simulink model "autopilota_v_15_last"  (R2022a)
settings: Solver=ode4  StartTime=0.0  StopTime=300  FixedStep=0.02  RelTol=1e-3
values from neighbouring files (symbols this model uses):
  attuatore_Amax = 20*(pi/180)    (= 0.349065850399)    [v2021_10_27_avvioSITL.m]    (also in v2021_10_27_calcoloAerodinamica.m)
  attuatore_Amin = -20*(pi/180)    (= -0.349065850399)    [v2021_10_27_avvioSITL.m]
  attuatore_Emax = 25*(pi/180)    (= 0.436332312999)    [v2021_10_27_avvioSITL.m]    (also in v2021_10_27_calcoloAerodinamica.m)
  attuatore_Emin = -25*(pi/180)    (= -0.436332312999)    [v2021_10_27_avvioSITL.m]
  attuatore_Rmax = 25*(pi/180)    (= 0.436332312999)    [v2021_10_27_avvioSITL.m]    (also in v2021_10_27_calcoloAerodinamica.m)
  attuatore_Rmin = -25*(pi/180)    (= -0.436332312999)    [v2021_10_27_avvioSITL.m]
  attuatore_Tmax = 0.99    [v2021_10_27_avvioSITL.m]
  attuatore_Tmin = 0    [v2021_10_27_avvioSITL.m]
  baccxINI = 0    [v2021_10_27_avvioSITL.m]
  baccyINI = 0    [v2021_10_27_avvioSITL.m]
  bacczINI = 0    [v2021_10_27_avvioSITL.m]
  bias = [baccxINI,baccyINI,bacczINI,bpINI,bqINI,brINI]    [v2021_10_27_avvioSITL.m]
  bpINI = 0    [v2021_10_27_avvioSITL.m]
  bqINI = 0    [v2021_10_27_avvioSITL.m]
  brINI = 0    [v2021_10_27_avvioSITL.m]
  final_h = 35    [v2021_10_27_avvioSITL.m]
  interventoA_05 = 20*0.8    (= 16)    [v2021_10_27_avvioSITL.m]
  interventoA_1 = 10    [v2021_10_27_avvioSITL.m]
  interventoE_05 = 25*0.8    (= 20)    [v2021_10_27_avvioSITL.m]
  interventoE_1 = 10    [v2021_10_27_avvioSITL.m]
  interventoT = 1*0.6    (= 0.6)    [v2021_10_27_avvioSITL.m]
  inv_A = 1    [v2021_10_27_avvioSITL.m]
  inv_comp_h = 1    [v2021_10_27_avvioSITL.m]
  inv_E = 1    [v2021_10_27_avvioSITL.m]
  inv_R = 1    [v2021_10_27_avvioSITL.m]
  inv_T = 1    [v2021_10_27_avvioSITL.m]
  K_AW_B_AP_quota = 1000    [v2021_10_27_avvioSITL.m]
  K_AW_B_becc = -250    [v2021_10_27_avvioSITL.m]
  K_AW_B_imb = 0    [v2021_10_27_avvioSITL.m]
  K_AW_B_roll = 500    [v2021_10_27_avvioSITL.m]
  K_imb_inv = -0.001306    [v2021_10_27_avvioSITL.m]
  Kd_AP_rotta = 0.995    [v2021_10_27_avvioSITL.m]
  Kd_h_app = 0.085    [v2021_10_27_avvioSITL.m]
  Kd_h_flare = 0.01    [v2021_10_27_avvioSITL.m]
  Ki_AP_quota_select = 0.01936    [v2021_10_27_avvioSITL.m]
  Ki_AP_rotta = 0.002    [v2021_10_27_avvioSITL.m]
  Ki_AP_vel = 0.025175    [v2021_10_27_avvioSITL.m]
  Ki_becch = -0.1963    [v2021_10_27_avvioSITL.m]
  Ki_h_app = 0.055    [v2021_10_27_avvioSITL.m]
  Ki_h_cruise = 0.008    [v2021_10_27_avvioSITL.m]
  Ki_h_flare = 0.07    [v2021_10_27_avvioSITL.m]
  Ki_roll = 0.004528    [v2021_10_27_avvioSITL.m]
  Kp_AP_quota_hold_h = 0.5503    [v2021_10_27_avvioSITL.m]
  Kp_AP_quota_hold_l = 0.5503    [v2021_10_27_avvioSITL.m]
  Kp_AP_quota_select = 0.02647    [v2021_10_27_avvioSITL.m]
  Kp_AP_rotta = 0.520    (= 0.52)    [v2021_10_27_avvioSITL.m]
  Kp_AP_vel = 0.132175    [v2021_10_27_avvioSITL.m]
  Kp_becch = -0.30    (= -0.3)    [v2021_10_27_avvioSITL.m]
  Kp_comp_h = 0.035    [v2021_10_27_avvioSITL.m]
  Kp_h_app_max = 0.086    [v2021_10_27_avvioSITL.m]
  Kp_h_app_min = 0.01    [v2021_10_27_avvioSITL.m]
  Kp_h_cruise = 0.04    [v2021_10_27_avvioSITL.m]
  Kp_h_flare = 0.1    [v2021_10_27_avvioSITL.m]
  Kp_imb = 0.0019415    [v2021_10_27_avvioSITL.m]
  Kp_p = 0.006913    [v2021_10_27_avvioSITL.m]
  Kp_q = -0.025    [v2021_10_27_avvioSITL.m]
  Kp_roll = 0.0718    [v2021_10_27_avvioSITL.m]
  Kp_Rotta_ATO = 4    [v2021_10_27_avvioSITL.m]
  Kp_Rotta_psi = -0.01    [v2021_10_27_avvioSITL.m]
  safe_phi = 55    [v2021_10_27_avvioSITL.m]
  safe_V = 40    [v2021_10_27_avvioSITL.m]
  Sensor_Offsets = [0,0,0]    [v2021_10_27_avvioSITL.m]
  theta_rot = 10    [v2021_10_27_avvioSITL.m]
  time_alarm_SAFE = 300    [v2021_10_27_avvioSITL.m]
  tsamp = 0.02    [v2021_10_27_avvioSITL.m]
  V_max = 35    [v2021_10_27_avvioSITL.m]
  V_stall = 15    [v2021_10_27_avvioSITL.m]
  vd_ini = 0    [v2021_10_27_avvioSITL.m]
  vel_wp1_al = 25    [v2021_10_27_avvioSITL.m]
  vel_wp2_al = 20    [v2021_10_27_avvioSITL.m]
undefined symbols (not defined in the file or in its folder): DiscIntNeverNeededParam, Newton, Q1B, R1B, Raphson, t_AP
libraries: simulink_extras x36, slpidlib x8, dspsigops x4, aerolibtransform2sys x2, aerolibtransform2 x2, cstblocks x1, simulink x1
(part 1 of 8)
settings Model: Creator=39339  LastModifiedBy=mvisc
settings SolverCC: AlgebraicLoopSolver=TrustRegion
settings DataIOCC: ReturnWorkspaceOutputs=off
settings DebuggingCC: ParameterPrecisionLossMsg=none  UnconnectedInputMsg=warning  UnconnectedOutputMsg=warning  UnconnectedLineMsg=warning  SFMachineParentedDataDiag=warning  ArithmeticOperatorsInVariantConditions=warning
settings ModelReferenceCC: ModelReferenceNumInstancesAllowed=Single
settings SFSimCC: SimUseLocalCustomCode=off  CustomCodeUndefinedFunction=UseInterfaceOnly
settings RTWCC: RTWUseLocalCustomCode=off  DLArmComputeVersion=19.05
settings CodeAppCC: StateflowObjectComments=on

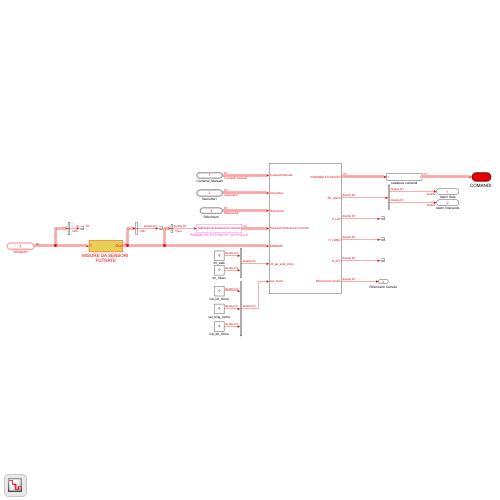
[thumbnail: Simulink's stored preview of the top-level diagram]
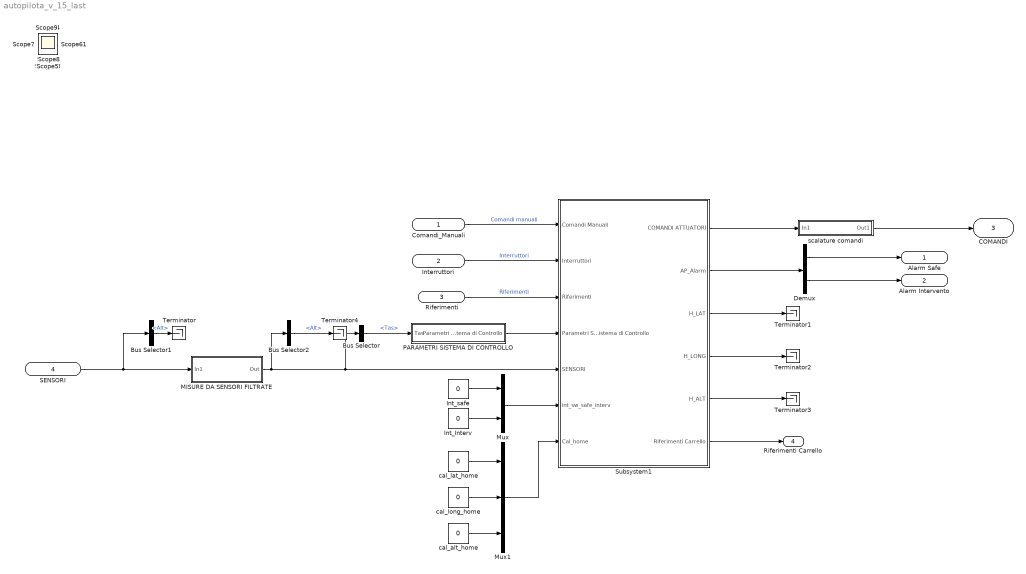
== system autopilota_v_15_last ==
  Comandi_Manuali : Inport  OutDataTypeStr=Bus: slBus4_manuali  SampleTime=[0.02,0]
  "Interruttori " : Inport  Port=2  OutDataTypeStr=Bus: slBus5_Interruttori  SampleTime=[0.02,0]
  Riferimenti : Inport  Port=3  OutDataTypeStr=Bus: slBus6_Riferimenti  SampleTime=[0.02,0]
  SENSORI : Inport  Port=4  OutDataTypeStr=Bus: slBus8_sensori2  SampleTime=[0.02,0]
  Bus Selector : BusSelector  OutputSignals=Tas
  Bus Selector1 : BusSelector  OutputSignals=Alt
  Bus Selector2 : BusSelector  OutputSignals=Alt
  Demux : Demux  Outputs=2
  Int_Interv : Constant  Value=0  SampleTime=t_AP
  Int_safe : Constant  Value=0  SampleTime=t_AP
  MISURE DA SENSORI FILTRATE : Subsystem
  Mux : Mux  Inputs=2
  Mux1 : Mux  Inputs=3
  PARAMETRI SISTEMA DI CONTROLLO : Subsystem
  Subsystem1 : Subsystem
  Terminator{,1..4} (5 alike) : Terminator
  cal_alt_home : Constant  Value=0  SampleTime=t_AP
  cal_lat_home : Constant  Value=0  SampleTime=t_AP
  cal_long_home : Constant  Value=0  SampleTime=t_AP
  "scalature comandi " : Subsystem
  Alarm Safe : Outport  OutDataTypeStr=double  PortDimensions=1  SampleTime=[0.02,0]  VectorParamsAs1DForOutWhenUnconnected=off
  Alarm Intervento : Outport  Port=2  OutDataTypeStr=double  PortDimensions=1  SampleTime=[0.02,0]  VectorParamsAs1DForOutWhenUnconnected=off
  "COMANDI " : Outport  Port=3  OutDataTypeStr=Bus: slBus8_comandi  SampleTime=[0.02,0]  VectorParamsAs1DForOutWhenUnconnected=off  LockScale=on
  Riferimenti Carrello : Outport  Port=4  VectorParamsAs1DForOutWhenUnconnected=off
  Scope{,1..11} (12 alike) : Scope
  wires:
  cal_long_home/1 -> Mux1/2
  Comandi_Manuali/1 -> Subsystem1/1(Comandi Manuali)  "Comandi manuali"
  Bus Selector/1 -> PARAMETRI SISTEMA DI CONTROLLO/1(Tas)  "<Tas>"
  "Interruttori "/1 -> Subsystem1/2("Interruttori ")  "Interruttori"
  PARAMETRI SISTEMA DI CONTROLLO/1(Parametri Sistema di Controllo) -> Subsystem1/4(Parametri Sistema di Controllo)
  Subsystem1/3(H_LAT) -> Terminator1/1
  Demux/1 -> Alarm Safe/1
  Subsystem1/5(H_ALT) -> Terminator3/1
  cal_lat_home/1 -> Mux1/1
  Int_safe/1 -> Mux/1
  Riferimenti/1 -> Subsystem1/3(Riferimenti)  "Riferimenti"
  Mux1/1 -> Subsystem1/7(Cal_home)
  cal_alt_home/1 -> Mux1/3
  Int_Interv/1 -> Mux/2
  Demux/2 -> Alarm Intervento/1
  Subsystem1/4(H_LONG) -> Terminator2/1
  Subsystem1/2(AP_Alarm) -> Demux/1
  Mux/1 -> Subsystem1/6(int_sw_safe_interv)
  SENSORI/1 -> MISURE DA SENSORI FILTRATE/1(In1), Bus Selector1/1
  MISURE DA SENSORI FILTRATE/1(Out) -> Bus Selector/1, Subsystem1/5(SENSORI), Bus Selector2/1
  "scalature comandi "/1(Out1) -> "COMANDI "/1
  Bus Selector2/1 -> Terminator4/1  "<Alt>"
  Bus Selector1/1 -> Terminator/1  "<Alt>"
  Subsystem1/6(Riferimenti Carrello) -> Riferimenti Carrello/1
  Subsystem1/1(COMANDI ATTUATORI) -> "scalature comandi "/1(In1)

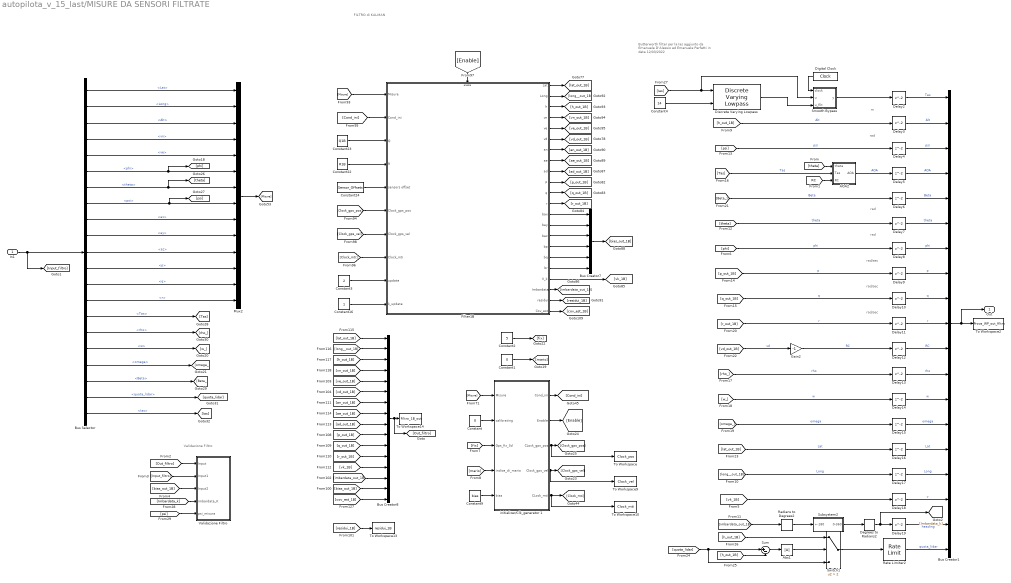
== system autopilota_v_15_last/MISURE DA SENSORI FILTRATE ==
  note: Validazione Filtro
  note: Butterworth filter per la Ias aggiunto da Emanuele D'Alessio ed Emanuele Perfetti in data 12/03/2022
  note: rad/sec
  note: rad/sec
  note: rad
  note: rad/sec
  note: FILTRO di KALMAN
  note: m
  note: rad
  note: rad
  In1 : Inport
  AOA2 : Subsystem
  Abs1 : Abs  SaturateOnIntegerOverflow=off
  Bus Creator1 : BusCreator  Inputs=19  OutDataTypeStr=Bus: slBus7_sensori
  Bus Creator7 : BusCreator  Inputs=6
  Bus Creator8 : BusCreator  Inputs=16
  Bus Selector : BusSelector  OutputSignals=Lat,Long,Alt,vn,ve,phi,theta,psi,ax,ay,az,p,q,r,Tas,rho,w,omega,Beta,quota_lidar,Ias
  Constant : Constant  Value=0
  Constant1 : Constant  Value=0
  Constant16 : Constant
  Constant2 : Constant  Value=5
  Constant22 : Constant  Value=R1B
  Constant23 : Constant  Value=Q1B
  Constant24 : Constant  Value=Sensor_Offsets
  Constant3 : Constant  Value=2
  Constant4 : Constant  Value=14
  Constant9 : Constant  Value=bias
  Degrees to Radians2 : simulink_extras/Transformations/Degrees to Radians
  Delay{2..19} (18 alike) : Delay
  Digital Clock : DigitalClock  SampleTime=0.02
  Discrete Varying Lowpass : cstblocks/Linear Parameter Varying/Discrete Varying Lowpass  N=2  w0=0  Ts=0.02
      settings: SourceProductBaseCode=CT
  Filter1B : Subsystem
  Gain2 : Gain  Gain=-1
  Mux2 : Mux  Inputs=14
  Radians to Degrees2 : simulink_extras/Transformations/Radians to Degrees
  Rate Limiter2 : RateLimiter  RisingSlewLimit=6  FallingSlewLimit=-6  SampleTimeMode=inherited
  Smooth Bypass : MATLAB Function  TreatAsAtomicUnit=on
  Subsystem2 : Subsystem
  Sum : Sum  Inputs=|+-
  Switch1 : Switch  Criteria=u2 > Threshold  Threshold=2  SaturateOnIntegerOverflow=off  InputSameDT=off
  To Workspace : ToWorkspace  VariableName=Clock_pos  SaveFormat=Timeseries  SampleTime=-1
  To Workspace10 : ToWorkspace  VariableName=Clock_mti  SaveFormat=Timeseries  SampleTime=-1
  To Workspace13 : ToWorkspace  VariableName=residui_1B  SaveFormat=Structure With Time  SampleTime=-1
  To Workspace14 : ToWorkspace  VariableName=Filtro_1B_out  SaveFormat=Timeseries  SampleTime=-1
  To Workspace2 : ToWorkspace  VariableName=Prova_WP_out_filtro  SaveFormat=Timeseries  SampleTime=-1
  To Workspace9 : ToWorkspace  VariableName=Clock_vel  SaveFormat=Timeseries  SampleTime=-1
  Validazione Filtro : Subsystem
  initializer/Clk_generator 1 : Subsystem
  Out : Outport  OutDataTypeStr=Bus: slBus7_sensori  VectorParamsAs1DForOutWhenUnconnected=off
  wires:
  Constant16/1 -> Filter1B/10(k_update)
  [Misure] -> initializer/Clk_generator 1/1(Misure)
  Delay14/1 -> Bus Creator1/13  "w"
  [Clock_gps_vel] -> Filter1B/7(Clock_gps_vel)
  Filter1B/21(residui) -> [residui_1B]
  Bus Selector/14 -> Mux2/14  "<r>"
  Filter1B/11(q) -> [q_out_1B]
  Filter1B/9(ad) -> [ad_out_1B]
  Filter1B/16(bp) -> Bus Creator7/4
  Gain2/1 -> Delay12/1  "RC"
  Filter1B/17(bq) -> Bus Creator7/5
  [long__out_1B] -> Bus Creator8/2
  [Clock_mti] -> Filter1B/8(Clock_mti)
  [mario] -> initializer/Clk_generator 1/4(indice_di_mario)
  Bus Creator7/1 -> [bias_out_1B]
  [h_out_1B] -> Bus Creator8/3
  [an_out_1B] -> Bus Creator8/7
  [Clock_gps_pos] -> Filter1B/6(Clock_gps_pos)
  Bus Selector/10 -> Mux2/10  "<ay>"
  [ad_out_1B] -> Bus Creator8/9
  Filter1B/5(ve) -> [ve_out_1B]
  Filter1B/3(h) -> [h_out_1B]
  [ae_out_1B] -> Bus Creator8/8
  Bus Creator8/1 -> [Out_filtro], To Workspace14/1
  Bus Selector/13 -> Mux2/13  "<q>"
  Constant3/1 -> Filter1B/9(update)
  [h_out_1B] -> Delay3/1  "Alt"
  Constant9/1 -> initializer/Clk_generator 1/5(bias)
  Filter1B/4(vn) -> [vn_out_1B]
  [lat_out_1B] -> Delay16/1  "Lat"
  [w_] -> Delay14/1  "w"
  Constant24/1 -> Filter1B/5(sensors offset)
  [Cond_ini] -> Filter1B/2(Cond_ini)
  Constant2/1 -> [fix]
  Filter1B/13(bax) -> Bus Creator7/1
  Filter1B/8(ae) -> [ae_out_1B]
  Filter1B/15(baz) -> Bus Creator7/3
  Delay19/1 -> Bus Creator1/18  "heading"
  [Misure] -> Filter1B/1(Misure)
  Delay9/1 -> Bus Creator1/8  "p"
  Filter1B/12(r) -> [r_out_1B]
  [vd_out_1B] -> Gain2/1  "vd"
  Filter1B/10(p) -> [p_out_1B]
  [cov_est_1B] -> Bus Creator8/16
  initializer/Clk_generator 1/5(CLock_mti) -> To Workspace10/1, [Clock_mti]
  Filter1B/6(vd) -> [vd_out_1B]
  Filter1B/22(Cov_est) -> [cov_est_1B]
  initializer/Clk_generator 1/2(Enable) -> [Enable]
  [vn_out_1B] -> Bus Creator8/4
  [imbardata_out_1B] -> Bus Creator8/14
  [vd_out_1B] -> Bus Creator8/6
  [Beta_] -> Delay6/1  "Beta"
  Delay6/1 -> Bus Creator1/5  "Beta"
  [rho_] -> Delay13/1  "rho"
  Mux2/1 -> [Misure]
  initializer/Clk_generator 1/4("Clock_gps_vel ") -> To Workspace9/1, [Clock_gps_vel]
  Delay4/1 -> Bus Creator1/3  "psi"
  [bias_out_1B] -> Bus Creator8/15
  Filter1B/18(br) -> Bus Creator7/6
  [ve_out_1B] -> Bus Creator8/5
  Constant/1 -> initializer/Clk_generator 1/2(calibrating)
  initializer/Clk_generator 1/3(CLock_gps_pos) -> To Workspace/1, [Clock_gps_pos]
  Delay15/1 -> Bus Creator1/14  "omega"
  Constant22/1 -> Filter1B/4(R)
  [p_out_1B] -> Delay9/1  "p"
  [phi] -> Delay8/1  "phi"
  Filter1B/2(Long) -> [long__out_1B]
  Bus Selector/5 -> Mux2/5  "<ve>"
  [lat_out_1B] -> Bus Creator8/1
  Bus Selector/15 -> [Tas]  "<Tas>"
  Delay18/1 -> Bus Creator1/17  "v"
  [q_out_1B] -> Bus Creator8/11
  Bus Selector/1 -> Mux2/1  "<Lat>"
  initializer/Clk_generator 1/1(Cond_ini) -> [Cond_ini]
  [fix] -> initializer/Clk_generator 1/3(Gps_fix_3d)
  Bus Selector/3 -> Mux2/3  "<Alt>"
  [p_out_1B] -> Bus Creator8/10
  Bus Selector/7 -> [theta], Mux2/7  "<theta>"
  [vk_1B] -> Bus Creator8/13
  Delay8/1 -> Bus Creator1/7  "phi"
  Filter1B/14(bay) -> Bus Creator7/2
  Delay12/1 -> Bus Creator1/11  "RC"
  Bus Creator1/1 -> Out/1, To Workspace2/1
  Delay5/1 -> Bus Creator1/4  "AOA"
  Constant1/1 -> [mario]
  Delay17/1 -> Bus Creator1/16  "Long"
  Constant23/1 -> Filter1B/3(Q)
  [r_out_1B] -> Delay11/1  "r"
  Bus Selector/8 -> Mux2/8, [psi]  "<psi>"
  Delay16/1 -> Bus Creator1/15  "Lat"
  [q_out_1B] -> Delay10/1  "q"
  Delay11/1 -> Bus Creator1/10  "r"
  [Tas] -> AOA2/2(Tas)  "Tas"
  [long__out_1B] -> Delay17/1  "Long"
  [Enable] -> Filter1B/Enable
  [imbardata_out_1B] -> Radians to Degrees2/1
  Filter1B/20(Imbardata) -> [imbardata_out_1B]
  Delay13/1 -> Bus Creator1/12  "rho"
  Filter1B/1(Lat) -> [lat_out_1B]
  Delay10/1 -> Bus Creator1/9  "q"
  Delay7/1 -> Bus Creator1/6  "theta"
  Delay3/1 -> Bus Creator1/2  "Alt"
  Filter1B/7(an) -> [an_out_1B]
  [omega_] -> Delay15/1  "omega"
  [theta] -> Delay7/1  "theta"
  Delay2/1 -> Bus Creator1/1  "Tas"
  AOA2/1(AOA) -> Delay5/1  "AOA"
  [residui_1B] -> To Workspace13/1
  [psi] -> Delay4/1  "psi"
  [r_out_1B] -> Bus Creator8/12
  [quota_lidar] -> Switch1/3, Sum/1
  [h_out_1B] -> Sum/2
  Sum/1 -> Abs1/1
  Abs1/1 -> Switch1/2
  [h_out_1B] -> Switch1/1
  Switch1/1 -> Rate Limiter2/1
  Rate Limiter2/1 -> Bus Creator1/19  "quota_lidar"
  In1/1 -> Bus Selector/1, [Input_filtro]
  Bus Selector/2 -> Mux2/2  "<Long>"
  Bus Selector/4 -> Mux2/4  "<vn>"
  Bus Selector/6 -> Mux2/6, [phi]  "<phi>"
  Bus Selector/9 -> Mux2/9  "<ax>"
  Bus Selector/11 -> Mux2/11  "<az>"
  Bus Selector/12 -> Mux2/12  "<p>"
  Bus Selector/16 -> [rho_]  "<rho>"
  Bus Selector/17 -> [w_]  "<w>"
  Bus Selector/18 -> [omega_]  "<omega>"
  Bus Selector/19 -> [Beta_]  "<Beta>"
  Bus Selector/20 -> [quota_lidar]  "<quota_lidar>"
  Filter1B/19(V_k) -> [vk_1B]
  Degrees to Radians2/1 -> Delay19/1, [Imbardata_k]
  Radians to Degrees2/1 -> Subsystem2/1(+-180)
  Subsystem2/1(0-360) -> Degrees to Radians2/1
  Bus Selector/21 -> [Ias]  "<Ias>"
  [Ias] -> Discrete Varying Lowpass/1, Smooth Bypass/2(u)
  Constant4/1 -> Discrete Varying Lowpass/2
  [theta] -> AOA2/1(theta)
  [RC] -> AOA2/3(RC)
  [Out_filtro] -> Validazione Filtro/1(Input)
  [Input_filtro] -> Validazione Filtro/2(Input1)
  [bias_out_1B] -> Validazione Filtro/3(Input2)
  [psi] -> Validazione Filtro/5(psi_misura)
  [Imbardata_k] -> Validazione Filtro/4(imbardata_K)
  [vk_1B] -> Delay18/1
  Discrete Varying Lowpass/1 -> Smooth Bypass/3(u_filt)
  Smooth Bypass/1(y) -> Delay2/1
  Digital Clock/1 -> Smooth Bypass/1(clock)

== system autopilota_v_15_last/PARAMETRI SISTEMA DI CONTROLLO ==
  Tas : Inport
  Bus Creator1 : BusCreator  Inputs=19
  K AntiWindup-Bumpless AP quota : Constant  Value=K_AW_B_AP_quota  OutDataTypeStr=single  SampleTime=t_AP
  K AntiWindup-Bumpless controllore beccheggio : Constant  Value=K_AW_B_becc  OutDataTypeStr=single  SampleTime=t_AP
  K AntiWindup-Bumpless controllore imbardata : Constant  Value=K_AW_B_imb  OutDataTypeStr=single  SampleTime=t_AP
  K AntiWindup-Bumpless controllore rollio : Constant  Value=K_AW_B_roll  OutDataTypeStr=single  SampleTime=t_AP
  K controllo imbardata inversa : Constant  Value=K_imb_inv  OutDataTypeStr=single  SampleTime=t_AP
  Ki AP quota Select : Constant  Value=Ki_AP_quota_select  OutDataTypeStr=single  SampleTime=t_AP
  Ki AP rotta1 : Constant  Value=Kd_AP_rotta  OutDataTypeStr=single  SampleTime=t_AP
  Ki AP velocità : Constant  Value=Ki_AP_vel  OutDataTypeStr=single  SampleTime=t_AP
  Ki controllore  beccheggio1 : Constant  Value=Ki_becch  OutDataTypeStr=single  SampleTime=t_AP
  Ki controllore  rollio3 : Constant  Value=Ki_roll  OutDataTypeStr=single  SampleTime=t_AP
  Kp AP quota Select : Constant  Value=Kp_AP_quota_select  OutDataTypeStr=single  SampleTime=t_AP
  Kp AP rotta : Constant  Value=Kp_AP_rotta  OutDataTypeStr=single  SampleTime=t_AP
  Kp AP velocità : Constant  Value=Kp_AP_vel  OutDataTypeStr=single  SampleTime=t_AP
  Kp controllore  rollio3 : Constant  Value=Kp_roll  OutDataTypeStr=single  SampleTime=t_AP
  Kp controllore  velocità rollio3 : Constant  Value=Kp_p  OutDataTypeStr=single  SampleTime=t_AP
  Kp controllore beccheggio1 : Constant  Value=Kp_becch  OutDataTypeStr=single  SampleTime=t_AP
  Kp controllore imbardata : Constant  Value=Kp_imb  OutDataTypeStr=single  SampleTime=t_AP
  Kp controllore velocità beccheggio1 : Constant  Value=Kp_q  OutDataTypeStr=single  SampleTime=t_AP
  Saturation : Saturate  UpperLimit=Kp_AP_quota_hold_h  LowerLimit=Kp_AP_quota_hold_l*0.9
  n-D Lookup Table : Lookup_n-D  NumberOfTableDimensions=1  BreakpointsForDimension1=[V_stall V_max*0.8]  Table=[Kp_AP_quota_hold_l Kp_AP_quota_hold_h]  RndMeth=Simplest
  Parametri Sistema di Controllo : Outport  VectorParamsAs1DForOutWhenUnconnected=off
  wires:
  Bus Creator1/1 -> Parametri Sistema di Controllo/1  "Cond.Volo.Richiesta"
  Kp controllore imbardata/1 -> Bus Creator1/7  "Kp_imb"
  Kp AP velocità/1 -> Bus Creator1/8  "Kp_AP_vel"
  Saturation/1 -> Bus Creator1/10  "Kp_AP_quota_hold"
  Kp AP quota Select/1 -> Bus Creator1/11  "Kp_AP_quota_select"
  Ki AP quota Select/1 -> Bus Creator1/12  "Ki_AP_quota_select"
  Kp AP rotta/1 -> Bus Creator1/13  "Kp_AP_rotta"
  K AntiWindup-Bumpless controllore beccheggio/1 -> Bus Creator1/15  "K_AW-B_becc"
  K AntiWindup-Bumpless controllore rollio/1 -> Bus Creator1/16  "K_AW-B_roll"
  K AntiWindup-Bumpless controllore imbardata/1 -> Bus Creator1/17  "K_AW-B_imb"
  K AntiWindup-Bumpless AP quota/1 -> Bus Creator1/18  "K_AW-B_AP_quota"
  Ki AP velocità/1 -> Bus Creator1/9  "Ki_AP_vel"
  Ki AP rotta1/1 -> Bus Creator1/14  "Ki_AP_rotta"
  Kp controllore  rollio3/1 -> Bus Creator1/4  "Kp_roll"
  Kp controllore  velocità rollio3/1 -> Bus Creator1/6  "Kp_p"
  Ki controllore  rollio3/1 -> Bus Creator1/5  "Ki_roll"
  n-D Lookup Table/1 -> Saturation/1
  Tas/1 -> n-D Lookup Table/1
  Kp controllore beccheggio1/1 -> Bus Creator1/1  "Kp_becch"
  Ki controllore  beccheggio1/1 -> Bus Creator1/2  "Ki_becch"
  Kp controllore velocità beccheggio1/1 -> Bus Creator1/3  "Kp_q"
  K controllo imbardata inversa/1 -> Bus Creator1/19  "K_imb_inv"

== system autopilota_v_15_last/Subsystem1 ==
  note: MODI A/P
  note: LOOP ESTERNI e SWITCH
  note: LOOP INTERNI e SWITCH
  note: SISTEMA DI GESTIONE
  Comandi Manuali : Inport
  "Interruttori " : Inport  Port=2
  Riferimenti : Inport  Port=3
  Parametri Sistema di Controllo : Inport  Port=4
  SENSORI : Inport  Port=5
  int_sw_safe_interv : Inport  Port=6
  Cal_home : Inport  Port=7
  AUTOPILOTI1 : Subsystem
  CONTROLLI INTERNI E SWITCH1 : Subsystem
  Demux : Demux  Outputs=2
  GESTIONE AUTOPILOTI1 : Subsystem
  Mux : Mux  Inputs=2
  Mux1 : Mux  Inputs=3
  Subsystem1 : Subsystem
  COMANDI ATTUATORI : Outport  VectorParamsAs1DForOutWhenUnconnected=off
  AP_Alarm : Outport  Port=2  VectorParamsAs1DForOutWhenUnconnected=off
  H_LAT : Outport  Port=3  VectorParamsAs1DForOutWhenUnconnected=off
  H_LONG : Outport  Port=4  VectorParamsAs1DForOutWhenUnconnected=off
  H_ALT : Outport  Port=5  VectorParamsAs1DForOutWhenUnconnected=off
  Riferimenti Carrello : Outport  Port=6  VectorParamsAs1DForOutWhenUnconnected=off
  wires:
  Subsystem1/2(Inner_loop_ATO) -> CONTROLLI INTERNI E SWITCH1/10(Inner_loop_ATO)
  Subsystem1/5(H_ALT) -> H_ALT/1
  [Switch_AL] -> CONTROLLI INTERNI E SWITCH1/8(Switch_AL)
  [Switch_ATO] -> CONTROLLI INTERNI E SWITCH1/7(Switch_ATO)
  Parametri Sistema di Controllo/1 -> CONTROLLI INTERNI E SWITCH1/1(Parametri Sistema di Controllo), AUTOPILOTI1/2(Parametri Sistema di Controllo)
  CONTROLLI INTERNI E SWITCH1/2(theta_track) -> AUTOPILOTI1/10(traking theta)
  Subsystem1/3(H_LAT) -> H_LAT/1
  Subsystem1/4(H_LONG) -> H_LONG/1
  CONTROLLI INTERNI E SWITCH1/1(Comandi Attuatori) -> COMANDI ATTUATORI/1
  Comandi Manuali/1 -> CONTROLLI INTERNI E SWITCH1/2(Comandi Manuali), AUTOPILOTI1/6(comandi), GESTIONE AUTOPILOTI1/3(Comandi Manuali)
  AUTOPILOTI1/2(Riferimenti Rollio e Beccheggio) -> CONTROLLI INTERNI E SWITCH1/6(Riferimenti Rollio e Beccheggio)
  GESTIONE AUTOPILOTI1/5(Alarm Safe) -> Mux/1, AUTOPILOTI1/5(Alarm Safe)
  Cal_home/1 -> Subsystem1/5(Cal_Home)
  GESTIONE AUTOPILOTI1/1(Switch Attuatori) -> Subsystem1/6(Switch_attuatori), CONTROLLI INTERNI E SWITCH1/4(Switch Attuatori), AUTOPILOTI1/7(Switch attuatori)
  Demux/1 -> GESTIONE AUTOPILOTI1/4(int_sw_safe)
  Demux/2 -> GESTIONE AUTOPILOTI1/5(int_sw_intervento)
  GESTIONE AUTOPILOTI1/4(Alarm Intervento) -> Mux/2
  Riferimenti/1 -> Subsystem1/3(waypoints e riferimenti vettoriali)
  GESTIONE AUTOPILOTI1/2(Riferimenti Safe) -> AUTOPILOTI1/4(Riferimenti Safe)
  SENSORI/1 -> GESTIONE AUTOPILOTI1/1(Sensori), Subsystem1/1(sensori), CONTROLLI INTERNI E SWITCH1/5(Sensori), AUTOPILOTI1/1(Sensori)
  Subsystem1/1(Riferimenti) -> CONTROLLI INTERNI E SWITCH1/9(riferimenti), AUTOPILOTI1/3(Riferimenti)
  GESTIONE AUTOPILOTI1/3(modo) -> Subsystem1/4(modo)
  int_sw_safe_interv/1 -> Demux/1
  [Switch_ATO] -> AUTOPILOTI1/8(Switch_ATO)
  GESTIONE AUTOPILOTI1/7(Switch_AL) -> [Switch_AL]
  AUTOPILOTI1/1(Riferimento Manetta) -> CONTROLLI INTERNI E SWITCH1/3(Riferimento Manetta)
  "Interruttori "/1 -> Subsystem1/2(Interruttori), GESTIONE AUTOPILOTI1/2("Interruttori ")
  Mux/1 -> AP_Alarm/1
  GESTIONE AUTOPILOTI1/6(Switch_ATO) -> [Switch_ATO]
  [Switch_AL] -> AUTOPILOTI1/9(Switch_AL)
  CONTROLLI INTERNI E SWITCH1/3(manetta_track) -> AUTOPILOTI1/11(manetta_track)
  CONTROLLI INTERNI E SWITCH1/4(track_phi) -> AUTOPILOTI1/12(track_phi)
  [Fase_ATO] -> Mux1/2  "Fase_ATO"
  Mux1/1 -> Riferimenti Carrello/1
  [modo] -> Mux1/1  "modo"
  [selector_AL] -> Mux1/3  "selector_AL"

== system autopilota_v_15_last/scalature comandi  ==
  note: 02/01/2022
      |
      | Abbiamo inserito un blocco "Cast to double"
      | dentro i blocchi: "THROTTLE1", "ELEVATOR1"
      | "AILERON1", ""RUDDER6"
  In1 : Inport
  AILERON1 : Subsystem
  Bus Creator : BusCreator  Inputs=4  OutDataTypeStr=Bus: slBus8_comandi
  Bus Selector : BusSelector  OutputSignals=Manetta,Equilibratore,Alettoni,Timone
  ELEVATOR1 : Subsystem
  RUDDER6 : Subsystem
  Radians to Degrees : simulink_extras/Transformations/Radians to Degrees
  Radians to Degrees1 : simulink_extras/Transformations/Radians to Degrees
  Radians to Degrees2 : simulink_extras/Transformations/Radians to Degrees
  THROTTLE1 : Subsystem
  Out1 : Outport  OutDataTypeStr=Bus: slBus8_comandi  VectorParamsAs1DForOutWhenUnconnected=off
  wires:
  Bus Creator/1 -> Out1/1
  ELEVATOR1/1(Out1) -> Bus Creator/2  "Equilibratore"
  RUDDER6/1(Out1) -> Bus Creator/4  "Timone"
  Bus Selector/4 -> Radians to Degrees2/1  "<Timone>"
  Bus Selector/1 -> THROTTLE1/1(In1)  "<Manetta>"
  Bus Selector/2 -> Radians to Degrees/1  "<Equilibratore>"
  Bus Selector/3 -> Radians to Degrees1/1  "<Alettoni>"
  THROTTLE1/1(Out1) -> Bus Creator/1  "Manetta"
  AILERON1/1(Out1) -> Bus Creator/3  "Alettoni"
  Radians to Degrees/1 -> ELEVATOR1/1(In1)
  Radians to Degrees1/1 -> AILERON1/1(In1)
  Radians to Degrees2/1 -> RUDDER6/1(In1)
  In1/1 -> Bus Selector/1

== system autopilota_v_15_last/MISURE DA SENSORI FILTRATE/AOA2 ==
  theta : Inport
  Tas : Inport  Port=2
  RC : Inport  Port=3
  Divide : Product  Inputs=*/
  Sum1 : Sum  Inputs=+-|
  Trigonometric Function : Trigonometry  Operator=asin
  AOA : Outport  VectorParamsAs1DForOutWhenUnconnected=off
  wires:
  RC/1 -> Divide/1
  Trigonometric Function/1 -> Sum1/2
  Tas/1 -> Divide/2
  Sum1/1 -> AOA/1
  Divide/1 -> Trigonometric Function/1
  theta/1 -> Sum1/1

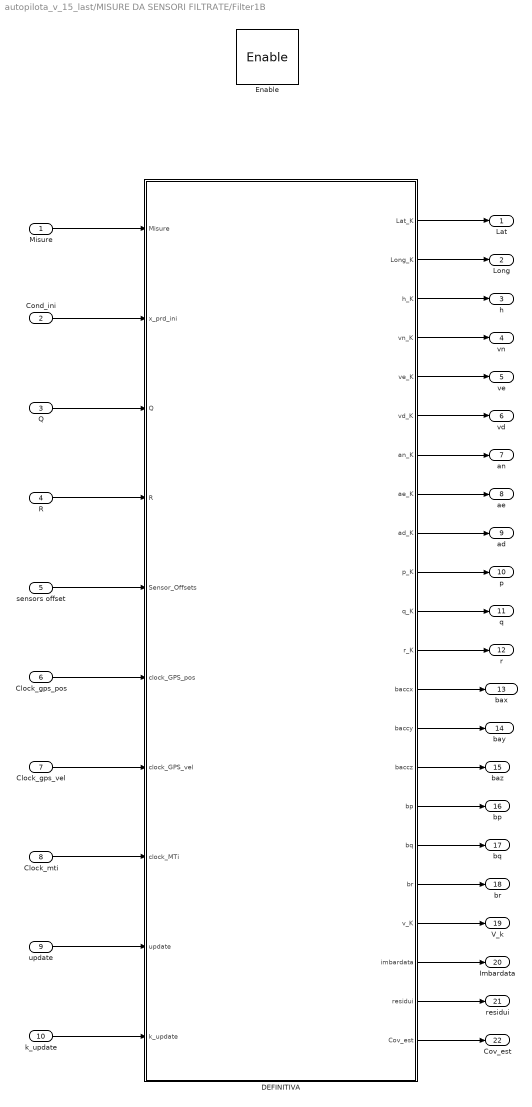
== system autopilota_v_15_last/MISURE DA SENSORI FILTRATE/Filter1B ==
  Misure : Inport
  Cond_ini : Inport  Port=2
  Q : Inport  Port=3
  R : Inport  Port=4
  sensors offset : Inport  Port=5
  Clock_gps_pos : Inport  Port=6
  Clock_gps_vel : Inport  Port=7
  Clock_mti : Inport  Port=8
  update : Inport  Port=9
  k_update : Inport  Port=10
  Enable : EnablePort
  DEFINITIVA : MATLAB Function  TreatAsAtomicUnit=on
  Lat : Outport  VectorParamsAs1DForOutWhenUnconnected=off
  Long : Outport  Port=2  VectorParamsAs1DForOutWhenUnconnected=off
  h : Outport  Port=3  VectorParamsAs1DForOutWhenUnconnected=off
  vn : Outport  Port=4  VectorParamsAs1DForOutWhenUnconnected=off
  ve : Outport  Port=5  VectorParamsAs1DForOutWhenUnconnected=off
  vd : Outport  Port=6  VectorParamsAs1DForOutWhenUnconnected=off
  an : Outport  Port=7  VectorParamsAs1DForOutWhenUnconnected=off
  ae : Outport  Port=8  VectorParamsAs1DForOutWhenUnconnected=off
  ad : Outport  Port=9  VectorParamsAs1DForOutWhenUnconnected=off
  p : Outport  Port=10  VectorParamsAs1DForOutWhenUnconnected=off
  q : Outport  Port=11  VectorParamsAs1DForOutWhenUnconnected=off
  r : Outport  Port=12  VectorParamsAs1DForOutWhenUnconnected=off
  bax : Outport  Port=13  VectorParamsAs1DForOutWhenUnconnected=off
  bay : Outport  Port=14  VectorParamsAs1DForOutWhenUnconnected=off
  baz : Outport  Port=15  VectorParamsAs1DForOutWhenUnconnected=off
  bp : Outport  Port=16  VectorParamsAs1DForOutWhenUnconnected=off
  bq : Outport  Port=17  VectorParamsAs1DForOutWhenUnconnected=off
  br : Outport  Port=18  VectorParamsAs1DForOutWhenUnconnected=off
  V_k : Outport  Port=19  VectorParamsAs1DForOutWhenUnconnected=off
  Imbardata : Outport  Port=20  VectorParamsAs1DForOutWhenUnconnected=off
  residui : Outport  Port=21  VectorParamsAs1DForOutWhenUnconnected=off
  Cov_est : Outport  Port=22  VectorParamsAs1DForOutWhenUnconnected=off
  wires:
  update/1 -> DEFINITIVA/9(update)
  Clock_mti/1 -> DEFINITIVA/8(clock_MTi)
  Clock_gps_vel/1 -> DEFINITIVA/7(clock_GPS_vel)
  sensors offset/1 -> DEFINITIVA/5(Sensor_Offsets)
  DEFINITIVA/5(ve_K) -> ve/1
  R/1 -> DEFINITIVA/4(R)
  Misure/1 -> DEFINITIVA/1(Misure)
  DEFINITIVA/2(Long_K) -> Long/1
  DEFINITIVA/1(Lat_K) -> Lat/1
  DEFINITIVA/4(vn_K) -> vn/1
  DEFINITIVA/3(h_K) -> h/1
  Q/1 -> DEFINITIVA/3(Q)
  DEFINITIVA/6(vd_K) -> vd/1
  Cond_ini/1 -> DEFINITIVA/2(x_prd_ini)
  Clock_gps_pos/1 -> DEFINITIVA/6(clock_GPS_pos)
  DEFINITIVA/7(an_K) -> an/1
  DEFINITIVA/8(ae_K) -> ae/1
  DEFINITIVA/9(ad_K) -> ad/1
  DEFINITIVA/10(p_K) -> p/1
  DEFINITIVA/11(q_K) -> q/1
  DEFINITIVA/12(r_K) -> r/1
  DEFINITIVA/13(baccx) -> bax/1
  DEFINITIVA/14(baccy) -> bay/1
  DEFINITIVA/15(baccz) -> baz/1
  DEFINITIVA/16(bp) -> bp/1
  DEFINITIVA/17(bq) -> bq/1
  DEFINITIVA/18(br) -> br/1
  DEFINITIVA/19(v_K) -> V_k/1
  DEFINITIVA/20(imbardata) -> Imbardata/1
  DEFINITIVA/21(residui) -> residui/1
  DEFINITIVA/22(Cov_est) -> Cov_est/1
  k_update/1 -> DEFINITIVA/10(k_update)

== system autopilota_v_15_last/MISURE DA SENSORI FILTRATE/Subsystem2 ==
  +-180 : Inport
  Constant : Constant  Value=360
  Gain : Gain  Gain=-1
  Sum : Sum  Inputs=|++
  Switch : Switch  Criteria=u2 > Threshold  SaturateOnIntegerOverflow=off  InputSameDT=off
  0-360 : Outport  VectorParamsAs1DForOutWhenUnconnected=off
  wires:
  Switch/1 -> 0-360/1
  Sum/1 -> Switch/1
  Gain/1 -> Switch/2
  +-180/1 -> Sum/1, Switch/3, Gain/1
  Constant/1 -> Sum/2

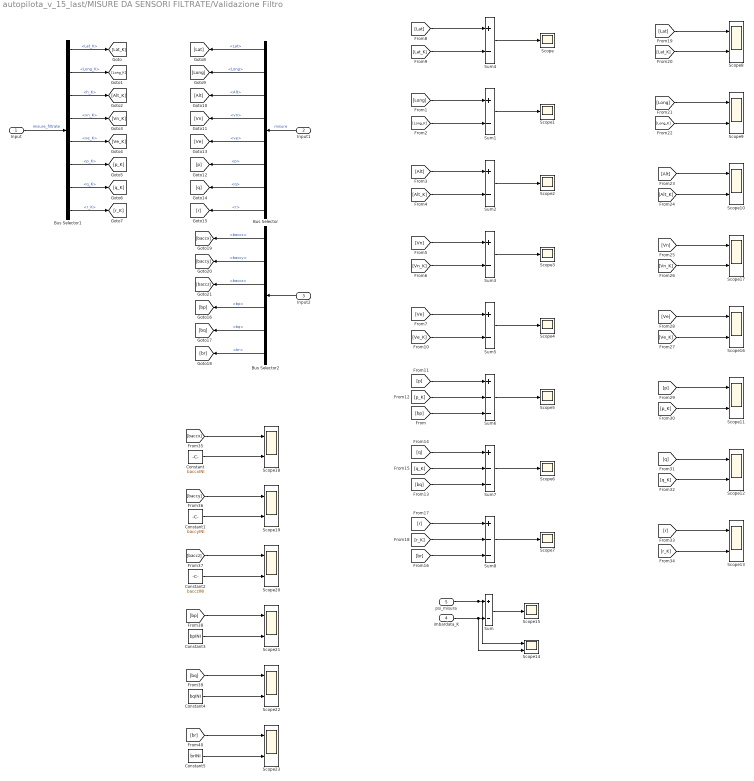
== system autopilota_v_15_last/MISURE DA SENSORI FILTRATE/Validazione Filtro ==
  Input : Inport
  Input1 : Inport  Port=2
  Input2 : Inport  Port=3
  imbardata_K : Inport  Port=4
  psi_misura : Inport  Port=5
  Bus Selector : BusSelector  OutputSignals=Lat,Long,Alt,vn,ve,p,q,r
  Bus Selector1 : BusSelector  OutputSignals=Lat_K,Long_K,h_K,vn_K,ve_K,p_K,q_K,r_K
  Bus Selector2 : BusSelector  OutputSignals=baccx,baccy,baccz,bp,bq,br
  Constant : Constant  Value=baccxINI
  Constant1 : Constant  Value=baccyINI
  Constant2 : Constant  Value=bacczINI
  Constant3 : Constant  Value=bpINI
  Constant4 : Constant  Value=bqINI
  Constant5 : Constant  Value=brINI
  Scope{,1..7,15} (9 alike) : Scope
  Scope{8..14,16..23} (15 alike) : Scope  NumInputPorts=2
  Sum{,1..5} (6 alike) : Sum  Inputs=+-
  Sum6 : Sum  Inputs=+--
  Sum7 : Sum  Inputs=+--
  Sum8 : Sum  Inputs=+--
  wires:
  Input/1 -> Bus Selector1/1  "misure_filtrate"
  Input1/1 -> Bus Selector/1  "misure"
  Input2/1 -> Bus Selector2/1
  Bus Selector1/3 -> [Alt_K]  "<h_K>"
  Bus Selector1/2 -> [Long_K]  "<Long_K>"
  Bus Selector1/1 -> [Lat_K]  "<Lat_K>"
  Bus Selector1/4 -> [Vn_K]  "<vn_K>"
  Bus Selector1/5 -> [Ve_K]  "<ve_K>"
  Bus Selector1/6 -> [p_K]  "<p_K>"
  Bus Selector1/7 -> [q_K]  "<q_K>"
  Bus Selector1/8 -> [r_K]  "<r_K>"
  Bus Selector/8 -> [r]  "<r>"
  Bus Selector/7 -> [q]  "<q>"
  Bus Selector/6 -> [p]  "<p>"
  Bus Selector/5 -> [Ve]  "<ve>"
  Bus Selector/4 -> [Vn]  "<vn>"
  Bus Selector/3 -> [Alt]  "<Alt>"
  Bus Selector/2 -> [Long]  "<Long>"
  Bus Selector/1 -> [Lat]  "<Lat>"
  Bus Selector2/6 -> [br]  "<br>"
  Bus Selector2/5 -> [bq]  "<bq>"
  Bus Selector2/4 -> [bp]  "<bp>"
  Bus Selector2/1 -> [baccx]  "<baccx>"
  Bus Selector2/2 -> [baccy]  "<baccy>"
  Bus Selector2/3 -> [baccz]  "<baccz>"
  [Lat] -> Sum4/1
  [Lat_K] -> Sum4/2
  [Long_K] -> Sum1/2
  [Long] -> Sum1/1
  [Alt_K] -> Sum2/2
  [Alt] -> Sum2/1
  [Vn_K] -> Sum3/2
  [Vn] -> Sum3/1
  [Ve_K] -> Sum5/2
  [Ve] -> Sum5/1
  [p_K] -> Sum6/2
  [p] -> Sum6/1
  [bp] -> Sum6/3
  [bq] -> Sum7/3
  [q_K] -> Sum7/2
  [q] -> Sum7/1
  [br] -> Sum8/3
  [r_K] -> Sum8/2
  [r] -> Sum8/1
  Sum4/1 -> Scope/1
  Sum1/1 -> Scope1/1
  Sum2/1 -> Scope2/1
  Sum3/1 -> Scope3/1
  Sum5/1 -> Scope4/1
  Sum6/1 -> Scope5/1
  Sum7/1 -> Scope6/1
  Sum8/1 -> Scope7/1
  psi_misura/1 -> Scope14/1, Sum/1
  imbardata_K/1 -> Scope14/2, Sum/2
  Sum/1 -> Scope15/1
  [Lat_K] -> Scope8/2
  [Lat] -> Scope8/1
  [Long] -> Scope9/1
  [Long_K] -> Scope9/2
  [Alt_K] -> Scope10/2
  [Alt] -> Scope10/1
  [Vn] -> Scope17/1
  [Vn_K] -> Scope17/2
  [Ve_K] -> Scope16/2
  [Ve] -> Scope16/1
  [p] -> Scope11/1
  [p_K] -> Scope11/2
  [q_K] -> Scope12/2
  [q] -> Scope12/1
  [r_K] -> Scope13/2
  [r] -> Scope13/1
  [baccz] -> Scope20/1
  [baccy] -> Scope19/1
  [baccx] -> Scope18/1
  [br] -> Scope23/1
  [bq] -> Scope22/1
  [bp] -> Scope21/1
  Constant5/1 -> Scope23/2
  Constant4/1 -> Scope22/2
  Constant3/1 -> Scope21/2
  Constant2/1 -> Scope20/2
  Constant1/1 -> Scope19/2
  Constant/1 -> Scope18/2

== system autopilota_v_15_last/MISURE DA SENSORI FILTRATE/initializer//Clk_generator 1 ==
  Misure : Inport
  calibrating : Inport  Port=2
  Gps_fix_3d : Inport  Port=3
  indice_di_mario : Inport  Port=4
  bias : Inport  Port=5
  Clock GPS1 : Subsystem
  Clock Mti : Subsystem
  Constant : Constant  Value=vd_ini
  Constant1 : Constant
  Constant2 : Constant
  In1 : InportShadow  Port=2
  MATLAB Function2 : MATLAB Function  TreatAsAtomicUnit=on
  Sample and Hold : dspsigops/Sample and Hold  Commented=on  trig=Rising edge  initCond=0  latchinput=off
  Scope : Scope
  Scope1 : Scope
  Switch : Switch  Criteria=u2 > Threshold  SaturateOnIntegerOverflow=off  InputSameDT=off
  Terminator : Terminator
  Cond_ini : Outport  VectorParamsAs1DForOutWhenUnconnected=off
  Enable : Outport  Port=2  VectorParamsAs1DForOutWhenUnconnected=off
  CLock_gps_pos : Outport  Port=3  VectorParamsAs1DForOutWhenUnconnected=off
  "Clock_gps_vel " : Outport  Port=4  VectorParamsAs1DForOutWhenUnconnected=off
  CLock_mti : Outport  Port=5  VectorParamsAs1DForOutWhenUnconnected=off
  wires:
  Gps_fix_3d/1 -> MATLAB Function2/5(fix)
  Clock GPS1/1(clk_pos) -> MATLAB Function2/3(clk_gps), CLock_gps_pos/1
  Clock Mti/1(Out1) -> CLock_mti/1, MATLAB Function2/2(clk_ahrs)
  Constant/1 -> MATLAB Function2/6(vd_ini)
  bias/1 -> MATLAB Function2/7(bias)
  indice_di_mario/1 -> Clock GPS1/1(In1)
  calibrating/1 -> MATLAB Function2/4(Calibrating)
  In1/1 -> Switch/3
  Constant1/1 -> Switch/1
  Switch/1 -> Enable/1
  Misure/1 -> Scope/1, MATLAB Function2/1(misure), Clock GPS1/2(In2), Clock Mti/1(In2)
  Clock GPS1/2(clk_vel) -> "Clock_gps_vel "/1
  MATLAB Function2/1(y) -> Cond_ini/1, Scope1/1
  MATLAB Function2/2(en) -> Terminator/1
  Constant2/1 -> Switch/2
  ? -> Sample and Hold/Trigger

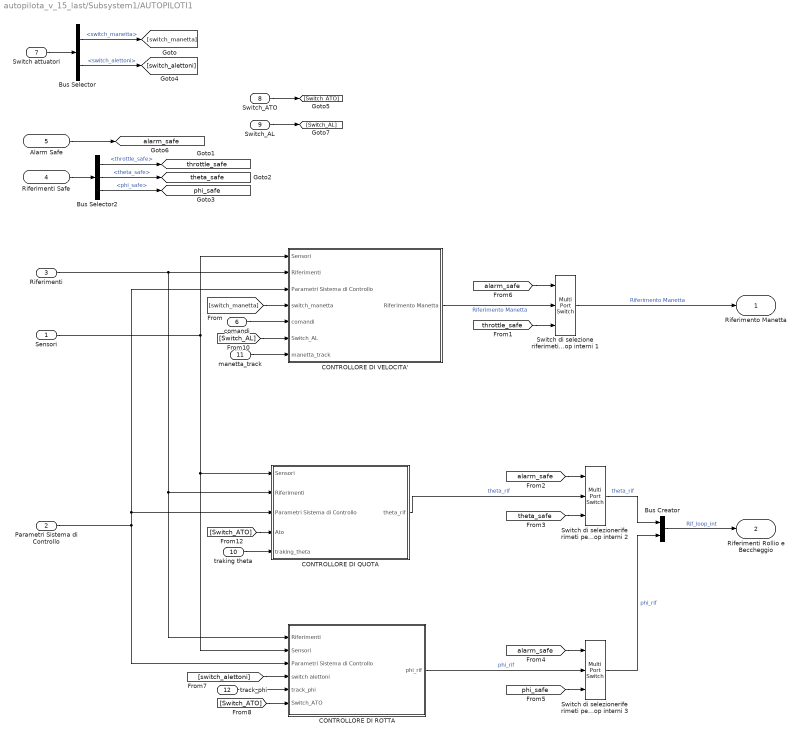
== system autopilota_v_15_last/Subsystem1/AUTOPILOTI1 ==
  Sensori : Inport
  Parametri Sistema di Controllo : Inport  Port=2
  Riferimenti : Inport  Port=3
  Riferimenti Safe : Inport  Port=4
  Alarm Safe : Inport  Port=5
  comandi : Inport  Port=6
  Switch attuatori : Inport  Port=7
  Switch_ATO : Inport  Port=8
  Switch_AL : Inport  Port=9
  traking theta : Inport  Port=10
  manetta_track : Inport  Port=11
  track_phi : Inport  Port=12
  Bus Creator : BusCreator  Inputs=2
  Bus Selector : BusSelector  OutputSignals=switch_manetta,switch_alettoni
  Bus Selector2 : BusSelector  OutputSignals=throttle_safe,theta_safe,phi_safe
  CONTROLLORE DI QUOTA : Subsystem
  CONTROLLORE DI ROTTA : Subsystem
  CONTROLLORE DI VELOCITA' : Subsystem
  Switch di selezione riferimeti per i loop interni 1 : MultiPortSwitch  DataPortOrder=Zero-based contiguous  Inputs=2  zeroidx=on  SaturateOnIntegerOverflow=off  InputSameDT=off
  Switch di selezioneriferimeti per i loop interni 2 : MultiPortSwitch  DataPortOrder=Zero-based contiguous  Inputs=2  zeroidx=on  SaturateOnIntegerOverflow=off  InputSameDT=off
  Switch di selezioneriferimeti per i loop interni 3 : MultiPortSwitch  DataPortOrder=Zero-based contiguous  Inputs=2  zeroidx=on  SaturateOnIntegerOverflow=off  InputSameDT=off
  Riferimento Manetta : Outport  VectorParamsAs1DForOutWhenUnconnected=off
  Riferimenti Rollio e Beccheggio : Outport  Port=2  VectorParamsAs1DForOutWhenUnconnected=off
  tag scope: alarm_safe=global, phi_safe=global, theta_safe=global, throttle_safe=global
  wires:
  Bus Creator/1 -> Riferimenti Rollio e Beccheggio/1  "Rif_loop_int"
  CONTROLLORE DI VELOCITA'/1(Riferimento Manetta) -> Switch di selezione riferimeti per i loop interni 1/2  "Riferimento Manetta"
  Switch di selezione riferimeti per i loop interni 1/1 -> Riferimento Manetta/1  "Riferimento Manetta"
  Switch di selezioneriferimeti per i loop interni 2/1 -> Bus Creator/1  "theta_rif"
  Switch di selezioneriferimeti per i loop interni 3/1 -> Bus Creator/2  "phi_rif"
  [alarm_safe] -> Switch di selezioneriferimeti per i loop interni 2/1
  [alarm_safe] -> Switch di selezioneriferimeti per i loop interni 3/1
  Sensori/1 -> CONTROLLORE DI VELOCITA'/1(Sensori), CONTROLLORE DI ROTTA/2(Sensori), CONTROLLORE DI QUOTA/1(Sensori)
  Riferimenti/1 -> CONTROLLORE DI ROTTA/1(Riferimenti), CONTROLLORE DI QUOTA/2(Riferimenti), CONTROLLORE DI VELOCITA'/2(Riferimenti)
  Parametri Sistema di Controllo/1 -> CONTROLLORE DI VELOCITA'/3(Parametri Sistema di Controllo), CONTROLLORE DI QUOTA/3(Parametri Sistema di Controllo), CONTROLLORE DI ROTTA/3(Parametri Sistema di Controllo)
  Riferimenti Safe/1 -> Bus Selector2/1
  Alarm Safe/1 -> [alarm_safe]
  Bus Selector2/1 -> [throttle_safe]  "<throttle_safe>"
  Bus Selector2/2 -> [theta_safe]  "<theta_safe>"
  Bus Selector2/3 -> [phi_safe]  "<phi_safe>"
  [alarm_safe] -> Switch di selezione riferimeti per i loop interni 1/1
  [throttle_safe] -> Switch di selezione riferimeti per i loop interni 1/3
  [theta_safe] -> Switch di selezioneriferimeti per i loop interni 2/3
  [phi_safe] -> Switch di selezioneriferimeti per i loop interni 3/3
  Switch attuatori/1 -> Bus Selector/1
  Bus Selector/1 -> [switch_manetta]  "<switch_manetta>"
  Bus Selector/2 -> [switch_alettoni]  "<switch_alettoni>"
  comandi/1 -> CONTROLLORE DI VELOCITA'/5(comandi)
  [switch_manetta] -> CONTROLLORE DI VELOCITA'/4(switch_manetta)
  [switch_alettoni] -> CONTROLLORE DI ROTTA/4("switch alettoni ")
  CONTROLLORE DI ROTTA/1(phi_rif) -> Switch di selezioneriferimeti per i loop interni 3/2  "phi_rif"
  Switch_ATO/1 -> [Switch_ATO]
  Switch_AL/1 -> [Switch_AL]
  [Switch_AL] -> CONTROLLORE DI VELOCITA'/6(Switch_AL)
  CONTROLLORE DI QUOTA/1(theta_rif) -> Switch di selezioneriferimeti per i loop interni 2/2  "theta_rif"
  [Switch_ATO] -> CONTROLLORE DI QUOTA/4(Ato)
  traking theta/1 -> CONTROLLORE DI QUOTA/5(traking_theta)
  manetta_track/1 -> CONTROLLORE DI VELOCITA'/7(manetta_track)
  track_phi/1 -> CONTROLLORE DI ROTTA/5(track_phi)
  [Switch_ATO] -> CONTROLLORE DI ROTTA/6(Switch_ATO)

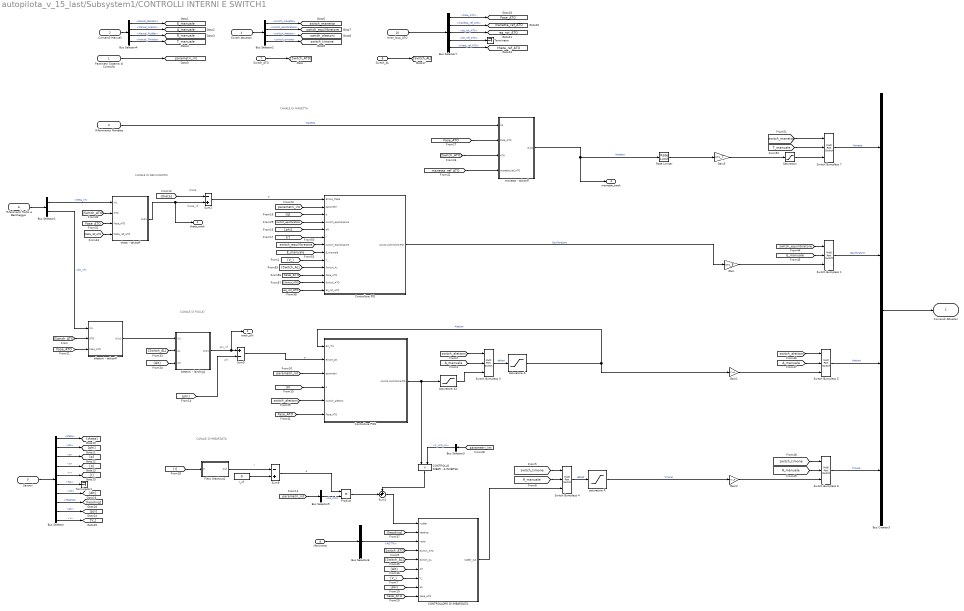
== system autopilota_v_15_last/Subsystem1/CONTROLLI INTERNI E SWITCH1 ==
  note: CANALE DI
      |  MANETTA
  note: theta
  note: theta_rif
  note: CANALE DI
      |  BECCHEGGIO
  note: CANALE
      | DI ROLLIO
  note: CANALE
      | DI IMBARDATA
  note: phi
  note: phi_rif
  note: r
  Parametri Sistema di Controllo : Inport
  Comandi Manuali : Inport  Port=2
  Riferimento Manetta : Inport  Port=3
  Switch Attuatori : Inport  Port=4
  Sensori : Inport  Port=5
  Riferimenti Rollio e Beccheggio : Inport  Port=6
  Switch_ATO : Inport  Port=7
  Switch_AL : Inport  Port=8
  riferimenti : Inport  Port=9
  Inner_loop_ATO : Inport  Port=10
  "  CONTROLLO IMBARDATA INVERSA" : Product  RndMeth=Zero
  Bus Creator3 : BusCreator  Inputs=4
  Bus Selector : BusSelector  OutputSignals=theta,phi,p,q,r,Tas,Alt,heading,psi,v
  Bus Selector1 : BusSelector  OutputSignals=theta_rif,phi_rif
  Bus Selector2 : BusSelector  OutputSignals=switch_manetta,switch_equilibratore,switch_alettoni,switch_timone
  Bus Selector3 : BusSelector  OutputSignals=K_imb_inv
  Bus Selector4 : BusSelector  OutputSignals=Manual_Elevator,Manual_Aileron,Manual_Rudder,Manual_Throttle
  Bus Selector5 : BusSelector  OutputSignals=Kp_imb
  Bus Selector6 : BusSelector  OutputSignals=ROTTA
  Bus Selector7 : BusSelector  OutputSignals=Fase_ATO,manetta_ref_ATO,eq_rot_ATO,phi_ref_ATO,theta_ref_ATO
  CONTROLLORE DI IMBARDATA : Subsystem
  Controllore PID : Subsystem
  Controllore PID1 : Subsystem
  Filtro Washout1 : Subsystem
  Gain : Gain  Gain=inv_E
  Gain1 : Gain  Gain=inv_A
  Gain2 : Gain  Gain=inv_R
  Gain3 : Gain  Gain=inv_T
  Product : Product  RndMeth=Zero
  Rate Limiter : RateLimiter  RisingSlewLimit=0.3  FallingSlewLimit=-0.3  SampleTimeMode=inherited
  Saturation : Saturate  UpperLimit=attuatore_Tmax  LowerLimit=attuatore_Tmin
  Sum1 : Sum  Inputs=++|
  Sum2 : Sum  Inputs=-+
  Sum5 : Sum  Inputs=+-
  Sum9 : Sum  Inputs=-+
  Switch Bumpless {1,3..7} (6 alike) : MultiPortSwitch  DataPortOrder=Zero-based contiguous  Inputs=2  zeroidx=on  SaturateOnIntegerOverflow=off  InputSameDT=off
  Terminator : Terminator
  Terminator1 : Terminator
  alettoni - landing1 : Subsystem
  alettoni - takeoff : Subsystem
  manetta - takeoff : Subsystem
  r_rif : Constant  Value=0  SampleTime=t_AP
  saturatore A : Saturate  UpperLimit=attuatore_Amax  LowerLimit=attuatore_Amin
  saturatore A1 : Saturate  UpperLimit=attuatore_Amax  LowerLimit=attuatore_Amin
  saturatore R : Saturate  UpperLimit=attuatore_Rmax  LowerLimit=attuatore_Rmin
  theta - takeoff : Subsystem
  Comandi Attuatori : Outport  VectorParamsAs1DForOutWhenUnconnected=off
  theta_track : Outport  Port=2  VectorParamsAs1DForOutWhenUnconnected=off
  manetta_track : Outport  Port=3  VectorParamsAs1DForOutWhenUnconnected=off
  track_phi : Outport  Port=4  VectorParamsAs1DForOutWhenUnconnected=off
  tag scope: A_manuale=global, E_manuale=global, Fase_ATO=global, R_manuale=global, T_manuale=global, eq_rot_ATO=global, manetta_ref_ATO=global, parametri_int=global, switch_alettoni=global, switch_equilibratore=global, switch_manetta=global, switch_timone=global, theta_ref_ATO=global
  wires:
  Comandi Manuali/1 -> Bus Selector4/1
  Bus Selector4/1 -> [E_manuale]  "<Manual_Elevator>"
  Bus Selector4/2 -> [A_manuale]  "<Manual_Aileron>"
  Bus Selector4/3 -> [R_manuale]  "<Manual_Rudder>"
  Bus Selector4/4 -> [T_manuale]  "<Manual_Throttle>"
  Parametri Sistema di Controllo/1 -> [parametri_int]
  Switch Attuatori/1 -> Bus Selector2/1
  Bus Selector2/1 -> [switch_manetta]  "<switch_manetta>"
  Bus Selector2/2 -> [switch_equilibratore]  "<switch_equilibratore>"
  Bus Selector2/3 -> [switch_alettoni]  "<switch_alettoni>"
  Bus Selector2/4 -> [switch_timone]  "<switch_timone>"
  Sensori/1 -> Bus Selector/1
  Riferimenti Rollio e Beccheggio/1 -> Bus Selector1/1
  Bus Selector1/2 -> alettoni - takeoff/1(In1)  "<phi_rif>"
  Switch Bumpless 3/1 -> saturatore A/1  "deltaA"
  saturatore A/1 -> Gain1/1, Controllore PID1/1(Err_Trk)  "Alettoni"
  [switch_alettoni] -> Switch Bumpless 3/1
  [A_manuale] -> Switch Bumpless 3/2
  [switch_timone] -> Switch Bumpless 4/1
  [R_manuale] -> Switch Bumpless 4/2
  r_rif/1 -> Sum9/2
  Filtro Washout1/1(Out) -> Sum9/1
  Bus Creator3/1 -> Comandi Attuatori/1
  Bus Selector3/1 -> "  CONTROLLO IMBARDATA INVERSA"/2  "<K_imb_inv>"
  [parametri_int] -> Bus Selector3/1
  Sum2/1 -> Controllore PID/1(Errore_theta)  "e"
  [switch_equilibratore] -> Controllore PID/4("switch_equilibratore ")
  saturatore A1/1 -> Switch Bumpless 3/3
  [parametri_int] -> Controllore PID/2(parametri)
  [parametri_int] -> Controllore PID1/3(parametri)
  Sum5/1 -> Controllore PID1/2(Errore_phi)  "e"
  Controllore PID1/1(Uscita controllore PID) -> "  CONTROLLO IMBARDATA INVERSA"/1, saturatore A1/1
  saturatore R/1 -> Gain2/1  "Timone"
  Switch Bumpless 4/1 -> saturatore R/1  "deltaR"
  Sum9/1 -> Product/1  "e"
  [parametri_int] -> Bus Selector5/1
  Bus Selector5/1 -> Product/2  "<Kp_imb>"
  Product/1 -> Sum1/2
  Sum1/1 -> CONTROLLORE DI IMBARDATA/1(rudder)
  "  CONTROLLO IMBARDATA INVERSA"/1 -> Sum1/1
  Switch_ATO/1 -> [Switch_ATO]
  Bus Selector/6 -> Terminator1/1  "<Tas>"
  Bus Selector/7 -> [Alt]  "<Alt>"
  alettoni - takeoff/1(Out1) -> alettoni - landing1/1(In1)
  [V_] -> CONTROLLORE DI IMBARDATA/7(V_)
  [Switch_ATO] -> CONTROLLORE DI IMBARDATA/4(Switch_ATO)
  CONTROLLORE DI IMBARDATA/1(rudder_out) -> Switch Bumpless 4/3
  Switch_AL/1 -> [Switch_AL]
  Controllore PID/1(Uscita controllore PID) -> Gain/1  "Equilibratore"
  alettoni - landing1/1(Out1) -> track_phi/1, Sum5/1
  [Switch_AL] -> alettoni - landing1/2(AL)
  [Alt] -> alettoni - landing1/3(Alt)
  [Switch_AL] -> CONTROLLORE DI IMBARDATA/5(Switch_AL)
  [Alt] -> CONTROLLORE DI IMBARDATA/6(Alt)
  riferimenti/1 -> Bus Selector6/1
  Bus Selector6/1 -> CONTROLLORE DI IMBARDATA/3(rotta)  "<ROTTA>"
  [heading] -> CONTROLLORE DI IMBARDATA/2(heading)
  Inner_loop_ATO/1 -> Bus Selector7/1
  Bus Selector7/1 -> [Fase_ATO]  "<Fase_ATO>"
  Bus Selector7/2 -> [manetta_ref_ATO]  "<manetta_ref_ATO>"
  Bus Selector7/3 -> [eq_rot_ATO]  "<eq_rot_ATO>"
  Bus Selector7/4 -> Terminator/1  "<phi_ref_ATO>"
  Bus Selector7/5 -> [theta_ref_ATO]  "<theta_ref_ATO>"
  manetta - takeoff/1(Out1) -> Rate Limiter/1, manetta_track/1  "Manetta"
  Riferimento Manetta/1 -> manetta - takeoff/1(In1)  "Manetta"
  [switch_alettoni] -> Controllore PID1/5("switch_alettoni ")
  [theta] -> Sum2/1
  Bus Selector/1 -> [theta]  "<theta>"
  [phi] -> Controllore PID/5("phi ")
  [phi] -> Sum5/2
  Bus Selector/2 -> [phi]  "<phi>"
  [p] -> Controllore PID1/4("p ")
  Bus Selector/3 -> [p]  "<p>"
  [q] -> Controllore PID/3("q ")
  Bus Selector/4 -> [q]  "<q>"
  [r] -> Controllore PID/6(r)
  [r] -> Filtro Washout1/1(In)
  Bus Selector/5 -> [r]  "<r>"
  Bus Selector/9 -> [psi]  "<psi>"
  [psi] -> CONTROLLORE DI IMBARDATA/8(psi)
  [Fase_ATO] -> CONTROLLORE DI IMBARDATA/9(Fase_ATO)
  [Switch_ATO] -> alettoni - takeoff/2(ATO)
  [Fase_ATO] -> alettoni - takeoff/3(Fase_ATO)
  [Switch_ATO] -> manetta - takeoff/3(ATO)
  [Fase_ATO] -> manetta - takeoff/2(Fase_ATO)
  [manetta_ref_ATO] -> manetta - takeoff/4(manetta_ref_ATO)
  Bus Selector1/1 -> theta - takeoff/1(In1)  "<theta_rif>"
  [Switch_ATO] -> theta - takeoff/2(ATO)
  [Fase_ATO] -> theta - takeoff/3(Fase_ATO)
  [Fase_ATO] -> Controllore PID1/6(Fase_ATO)
  Bus Selector/8 -> [heading]  "<heading>"
  [theta_ref_ATO] -> theta - takeoff/4(theta_ref_ATO)
  Bus Selector/10 -> [V_]  "<v>"
  theta - takeoff/1(Out1) -> theta_track/1, Sum2/2
  Switch Bumpless 1/1 -> Bus Creator3/2  "Equilibratore"
  [E_manuale] -> Switch Bumpless 1/2
  [switch_equilibratore] -> Switch Bumpless 1/1
  Gain/1 -> Switch Bumpless 1/3
  [switch_alettoni] -> Switch Bumpless 5/1
  [A_manuale] -> Switch Bumpless 5/2
  Switch Bumpless 5/1 -> Bus Creator3/3  "Alettoni"
  Gain1/1 -> Switch Bumpless 5/3
  [switch_timone] -> Switch Bumpless 6/1
  [R_manuale] -> Switch Bumpless 6/2
  Switch Bumpless 6/1 -> Bus Creator3/4  "Timone"
  Gain2/1 -> Switch Bumpless 6/3
  [switch_manetta] -> Switch Bumpless 7/1
  [T_manuale] -> Switch Bumpless 7/2
  Switch Bumpless 7/1 -> Bus Creator3/1  "Manetta"
  Gain3/1 -> Saturation/1
  [switch_equilibratore] -> Controllore PID/7(switch_equilibratore)
  [E_manuale] -> Controllore PID/8(E_manuale)
  [Switch_AL] -> Controllore PID/10(Switch_AL)
  [V_] -> Controllore PID/9(V_)
  [Fase_ATO] -> Controllore PID/11(Fase_ATO)
  [Switch_ATO] -> Controllore PID/12(Switch_ATO)
  [eq_rot_ATO] -> Controllore PID/13(Eq_rot_ATO)
  Rate Limiter/1 -> Gain3/1
  Saturation/1 -> Switch Bumpless 7/3
